simulink library "ddm"  (R2021b)
settings: Solver=VariableStepAuto  StartTime=0.0  StopTime=10.0  RelTol=1e-3
undefined symbols (not defined in the file or in its folder): ENUM_ADASACCSTA_ERROR, ENUM_ADASACCSTA_OFF, ENUM_ADASACCSTA_STANDBY, ENUM_ADASISASTA_OFF, ENUM_ALLOWMOV_ALLOWREADY, ENUM_APS, ENUM_BRKSTA_ERROR, ENUM_BRKSTA_OFF, ENUM_BRKSTA_ON, ENUM_BRKSW_INVALID, ENUM_BRKSW_OFF, ENUM_BRKSW_ON, ENUM_CHGPREACTERRSTA_OBCPRE, ENUM_DCDCFAULTSTA_ANYFAULTLV1, ENUM_DCDCFAULTSTA_ANYFAULTLV2, ENUM_DRIVETRAIN_AWD, ENUM_DRIVETRAIN_FWD, ENUM_DRIVETRAIN_RWD, ENUM_DRSEATSTA_INVALID, ENUM_EDUDRTSTA_NORMAL, ENUM_EPBSTA_APPLIED, ENUM_EPBSTA_RELEASED, ENUM_HVBATTREADYPRE_READY, ENUM_MCUWARN_LV0, ENUM_MCUWARN_LV1, ENUM_MCUWARN_LV2, ENUM_MCUWARN_LV3, ENUM_MCUWARN_NOERROR, ENUM_OBCFAULTSTA_ANYFAULT, ENUM_PAS_R2F2, ENUM_PDFAULT_BATTPDFAIL, ENUM_PDFAULT_DCDCDISABLE, ENUM_PDFAULT_MCUDISABLE, ENUM_PDFAULT_MCUDISCHRG, ENUM_POWERSTA_OFF, ENUM_POWERSTA_ON, ENUM_POWERSTA_READY, ENUM_POWERSTA_STANDBY, ENUM_PRESSINDI_LOW, ENUM_PUFAULT_BATTUPFAIL, ENUM_PUFAULT_DCDCENABLEFAIL, ENUM_PUFAULT_PRECHRGCHKFAIL, ENUM_PUFAULT_SAFETYCHKFAIL, ENUM_PUSTATE_COMPLETED, ENUM_PWRSTASW_OFF, ENUM_PWRSTASW_OFFA, ENUM_PWRSTASW_OFFCHVCHRG, ENUM_PWRSTASW_OFFCLVCHRG, ENUM_PWRSTASW_ON, ENUM_PWRSTASW_ONHVCHRG, ENUM_PWRSTASW_READY, ENUM_PWRSTASW_STANDBY, ENUM_RANGESTA_12IN, ENUM_SHIFTCOMMAND_D, ENUM_SHIFTCOMMAND_N, ENUM_SHIFTCOMMAND_P, ENUM_SHIFTCOMMAND_R, ENUM_VEHMALFUNLV_2ND, ENUM_VEHMALFUNLV_3RD, ENUM_VEHMALFUNLV_4TH ... (+835)
libraries: hcu_lib x750, $bdroot x12, simulink x5
(part 13 of 28)

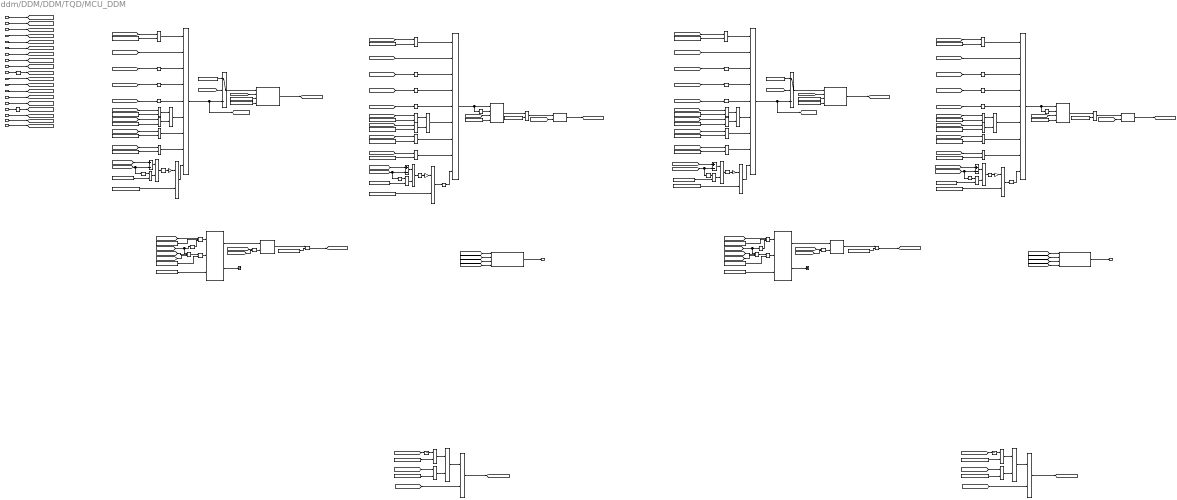
== system ddm/DDM/DDM/TQD/MCU_DDM ==
  note: Front Motor Torque Response Error (FrMCUTqErr)
  note: Fail Safe During Detection
  note: Test Pass Creteria
  note: Test Dtection Criteria
  note: Fail Safe After Detection
  note: Fail Safe During Detection
  note: Test Pass Creteria
  note: Rear Motor Torque Response Error (RrMCUTqErr)
  note: Test Dtection Criteria
  note: Fail Safe After Detection
  task_time_s : Inport
  VPMM_SysPwrSta_enum : Inport  Port=2
  No_CAN3_BUS_OFF : Inport  Port=3
  VDDM_MCUF1NoComCFS_flg : Inport  Port=4
  VDDM_MCUF1RCErrCFS_flg : Inport  Port=5
  VDDM_MCUF1CSErrCFS_flg : Inport  Port=6
  VINP_VehSpeed_kph : Inport  Port=7
  VINP_FrEDUDrtSta_flg : Inport  Port=8
  VINP_FrEDURealTMTq_Nm : Inport  Port=9
  VTQR_FrTMTqReq_Nm : Inport  Port=10
  VDDM_MCUR1NoComCFS_flg : Inport  Port=11
  VDDM_MCUR1RCErrCFS_flg : Inport  Port=12
  VDDM_MCUR1CSErrCFS_flg : Inport  Port=13
  VINP_RrEDUDrtSta_flg : Inport  Port=14
  VINP_RrEDURealTMTq_Nm : Inport  Port=15
  VTQR_RrTMTqReq_Nm : Inport  Port=16
  VINP_MCUWarnF_enum : Inport  Port=17
  VINP_MCUWarnR_enum : Inport  Port=18
  DTC_clear_request : Inport  Port=19
  Abs{,1..7} (8 alike) : Abs
  Add{,1..3} (4 alike) : Sum  Inputs=+-
  Constant{,1,47..48} (4 alike) : Constant  Value=eps
  Constant10 : Constant  Value=ENUM_POWERSTA_OFF
  Constant11 : Constant  Value=ENUM_POWERSTA_STANDBY
  Constant12 : Constant  Value=KDDM_RrMCUTqErrDetSW_flg
  Constant13 : Constant  Value=KDDM_FrMCUTqErrDetSW_flg
  Constant14 : Constant  Value=KDDM_FrMCUTqErrPassSW_flg
  Constant15 : Constant  Value=KDDM_FrMCUTqErrDet_pct
  Constant{4,16,26,32} (4 alike) : Constant  Value=ENUM_MCUWARN_LV0
  Constant{17,27,33,44} (4 alike) : Constant  Value=ENUM_PWRSTASW_OFF
  Constant18 : Constant  Value=ENUM_POWERSTA_OFF
  Constant19 : Constant  Value=ENUM_POWERSTA_STANDBY
  Constant2 : Constant  Value=KDDM_FrMCUTqErrCFSSW_flg
  Constant{5,20,29,34} (4 alike) : Constant  Value=ENUM_MCUWARN_NOERROR
  Constant{6,21,30,35} (4 alike) : Constant  Value=ENUM_EDUDRTSTA_NORMAL
  Constant22 : Constant  Value=KDDM_RrMCUTqErrPassSW_flg
  Constant23 : Constant  Value=KDDM_RrMCUTqErrCFSSW_flg
  Constant24 : Constant  Value=FALSE
  Constant25 : Constant  Value=KDDM_RrMCUTqErrDet_pct
  Constant28 : Constant  Value=KDDM_RrMCUTqErrDTC_cnt
  Constant3 : Constant  Value=KDDM_FrMCUTqErrDet_kph
  Constant31 : Constant  Value=KDDM_RrMCUTqErrDet_kph
  Constant36 : Constant  Value=KDDM_RrMCUTqErrPassTO_s
  Constant37 : Constant  Value=KDDM_RrMCUTqErrDetTO_s
  Constant38 : Constant  Value=KDDM_RrMCUTqErrDet_kph
  Constant39 : Constant  Value=KDDM_RrMCUTqErrPassTO_s
  Constant40 : Constant  Value=KDDM_RrMCUTqErrDTC_cnt
  Constant41 : Constant  Value=KDDM_FrMCUTqErrDet_pct
  Constant42 : Constant  Value=FALSE
  Constant43 : Constant  Value=KDDM_FrMCUTqErrDTC_cnt
  Constant45 : Constant  Value=KDDM_FrMCUTqErrPassTO_s
  Constant46 : Constant  Value=KDDM_FrMCUTqErrDetTO_s
  Constant7 : Constant  Value=KDDM_FrMCUTqErrDet_kph
  Constant70 : Constant  Value=KDDM_FrMCUTqErrPassTO_s
  Constant8 : Constant  Value=KDDM_FrMCUTqErrDTC_cnt
  Constant9 : Constant  Value=KDDM_RrMCUTqErrDet_pct
  DTC_Couter1 : hcu_lib/Basic_Blocks/DTC_Couter
  DTC_Couter2 : hcu_lib/Basic_Blocks/DTC_Couter
  DTC_Info : hcu_lib/Basic_Blocks/DTC_Info
  DTC_Info1 : hcu_lib/Basic_Blocks/DTC_Info
  Divide{,1..3} (4 alike) : Product  Inputs=*/
  Equal{1,3..4,6..10,15..16,21..22,30..31,33..34} (16 alike) : RelationalOperator  Operator===  OutDataTypeStr=boolean  RndMeth=Simplest
  Equal{5,11..12,17..18,27} (6 alike) : RelationalOperator  OutDataTypeStr=boolean  RndMeth=Simplest
  Equal{2,13,19,23} (4 alike) : RelationalOperator  Operator=>  OutDataTypeStr=boolean  RndMeth=Simplest
  Equal{14,20,24,26} (4 alike) : RelationalOperator  Operator=~=  OutDataTypeStr=boolean  RndMeth=Simplest
  Gain{,1..3} (4 alike) : Gain  Gain=100  OutDataTypeStr=single
  Logical Operator{1..2,12,16,20,25,38,40} (8 alike) : Logic  Operator=OR  AllPortsSameDT=off  OutDataTypeStr=boolean
  Logical Operator{3,7,9..10,13..15,17,21..23,26,28,34..37,39} (18 alike) : Logic  Operator=NOT  AllPortsSameDT=off  OutDataTypeStr=boolean
  Logical Operator{11,18,27,30} (4 alike) : Logic  Inputs=9  AllPortsSameDT=off  OutDataTypeStr=boolean
  Logical Operator{4,8,19,24,29,33} (6 alike) : Logic  AllPortsSameDT=off  OutDataTypeStr=boolean
  Logical Operator31 : Logic  Operator=OR  Inputs=3  AllPortsSameDT=off  OutDataTypeStr=boolean
  Logical Operator32 : Logic  Inputs=3  AllPortsSameDT=off  OutDataTypeStr=boolean
  Logical Operator5 : Logic  Operator=OR  Inputs=3  AllPortsSameDT=off  OutDataTypeStr=boolean
  Logical Operator6 : Logic  Inputs=3  AllPortsSameDT=off  OutDataTypeStr=boolean
  Max{,1..3} (4 alike) : MinMax  Function=max  Inputs=2
  Round : Rounding  Operator=round
  Round1 : Rounding  Operator=round
  SR_Latch{1..3,12} (4 alike) : hcu_lib/Basic_Blocks/SR_Latch
  Switch1 : Switch  Criteria=u2 ~= 0
  Switch6 : Switch  Criteria=u2 ~= 0
  Terminator : Terminator
  Terminator1 : Terminator
  Test Detection Criteria1 : hcu_lib/Basic_Blocks/Test Detection Criteria
  Test Detection Criteria2 : hcu_lib/Basic_Blocks/Test Detection Criteria
  Timer1 : hcu_lib/Basic_Blocks/Timer
  Timer2 : hcu_lib/Basic_Blocks/Timer
  Unit Delay : UnitDelay  SampleTime=-1  HasFrameUpgradeWarning=on
  Unit Delay1 : UnitDelay  SampleTime=-1  HasFrameUpgradeWarning=on
  VDDM_FrMCUTqErrDTC_raw32 : Outport
  VDDM_RrMCUTqErrDTC_raw32 : Outport  Port=2
  wires:
  Equal26/1 -> Logical Operator30/1
  Constant44/1 -> Equal26/2
  [VPMM_SysPwrSta_enum] -> Equal26/1
  Logical Operator12/1 -> [VDDM_FrMCUTqErrCFSRls_flg]  "VDDM_FrMCUTqErrCFSRls_flg"
  Constant11/1 -> Equal4/2
  [VPMM_SysPwrSta_enum] -> Unit Delay/1
  [DTC_clear_request] -> Logical Operator12/2
  Equal3/1 -> Logical Operator4/1
  [VPMM_SysPwrSta_enum] -> Equal4/1
  [No_CAN_BUS_OFF] -> Logical Operator30/2
  Equal4/1 -> Logical Operator4/2
  Unit Delay/1 -> Equal3/1
  Logical Operator4/1 -> Logical Operator12/1
  Constant10/1 -> Equal3/2
  Constant3/1 -> Equal2/2
  [VINP_VehSpeed_kph] -> Equal2/1
  Constant4/1 -> Equal6/2
  Constant5/1 -> Equal7/2
  Equal6/1 -> Logical Operator1/1
  Equal7/1 -> Logical Operator1/2
  Logical Operator1/1 -> Logical Operator30/6
  [VINP_FrEDUDrtSta_flg] -> Equal10/1
  Constant6/1 -> Equal10/2
  Equal10/1 -> Logical Operator30/7
  Equal2/1 -> Logical Operator30/8
  [VDDM_MCUF1CSErrCFS_flg] -> Logical Operator10/1
  [VDDM_MCUF1RCErrCFS_flg] -> Logical Operator9/1
  Logical Operator9/1 -> Logical Operator30/4
  [VDDM_MCUF1NoComCFS_flg] -> Logical Operator7/1
  Logical Operator7/1 -> Logical Operator30/3
  Logical Operator10/1 -> Logical Operator30/5
  Add/1 -> Divide/1
  Abs/1 -> Gain/1
  Divide/1 -> Abs/1
  [VINP_FrEDURealTMTq_Nm] -> Add/1
  [VTQR_FrTMTqReq_Nm] -> Abs4/1, Add/2
  Gain/1 -> Equal12/1
  Equal12/1 -> Logical Operator30/9
  Constant15/1 -> Equal12/2
  Logical Operator2/1 -> Logical Operator11/6
  [VINP_FrEDUDrtSta_flg] -> Equal1/1
  Constant20/1 -> Equal16/2
  [VDDM_MCUF1NoComCFS_flg] -> Logical Operator13/1
  Equal1/1 -> Logical Operator11/7
  Constant16/1 -> Equal15/2
  Equal13/1 -> Logical Operator11/8
  Logical Operator14/1 -> Logical Operator11/4
  [VDDM_MCUF1RCErrCFS_flg] -> Logical Operator14/1
  Constant7/1 -> Equal13/2
  Constant21/1 -> Equal1/2
  [VINP_VehSpeed_kph] -> Equal13/1
  Logical Operator3/1 -> Logical Operator11/5
  [VDDM_MCUF1CSErrCFS_flg] -> Logical Operator3/1
  Constant17/1 -> Equal14/2
  [No_CAN_BUS_OFF] -> Logical Operator11/2
  Equal16/1 -> Logical Operator2/2
  [VPMM_SysPwrSta_enum] -> Equal14/1
  Equal14/1 -> Logical Operator11/1
  Equal15/1 -> Logical Operator2/1
  Logical Operator13/1 -> Logical Operator11/3
  Equal11/1 -> Logical Operator15/1
  Logical Operator15/1 -> Logical Operator11/9
  [VDDM_MCUR1CSErrCFS_flg] -> Logical Operator17/1
  Equal8/1 -> Logical Operator18/7
  Logical Operator22/1 -> Logical Operator18/4
  [VDDM_MCUR1RCErrCFS_flg] -> Logical Operator22/1
  Equal33/1 -> Logical Operator16/1
  [VINP_MCUWarnR_enum] -> Equal33/1
  [VINP_VehSpeed_kph] -> Equal23/1
  Constant38/1 -> Equal19/2
  [VDDM_MCUR1CSErrCFS_flg] -> Logical Operator26/1
  Constant27/1 -> Equal20/2
  Logical Operator21/1 -> Logical Operator18/3
  Equal21/1 -> Logical Operator25/1
  Logical Operator26/1 -> Logical Operator18/5
  [VINP_VehSpeed_kph] -> Equal19/1
  Constant18/1 -> Equal30/2
  [VPMM_SysPwrSta_enum] -> Equal20/1
  [No_CAN_BUS_OFF] -> Logical Operator18/2
  Logical Operator23/1 -> Logical Operator18/9
  Logical Operator29/1 -> Logical Operator20/1
  Equal20/1 -> Logical Operator18/1
  [VINP_MCUWarnR_enum] -> Equal34/1
  Logical Operator17/1 -> Logical Operator27/5
  Equal34/1 -> Logical Operator16/2
  Equal31/1 -> Logical Operator29/2
  [VPMM_SysPwrSta_enum] -> Equal31/1
  Equal18/1 -> Logical Operator27/9
  [VDDM_MCUR1NoComCFS_flg] -> Logical Operator35/1
  Equal22/1 -> Logical Operator25/2
  Constant33/1 -> Equal24/2
  Equal23/1 -> Logical Operator27/8
  Constant26/1 -> Equal21/2
  Equal19/1 -> Logical Operator18/8
  Equal9/1 -> Logical Operator27/7
  Unit Delay1/1 -> Equal30/1
  [VDDM_MCUR1RCErrCFS_flg] -> Logical Operator37/1
  Constant30/1 -> Equal8/2
  Constant29/1 -> Equal22/2
  [VDDM_MCUR1NoComCFS_flg] -> Logical Operator21/1
  Constant35/1 -> Equal9/2
  Logical Operator35/1 -> Logical Operator27/3
  Constant32/1 -> Equal33/2
  [VINP_RrEDUDrtSta_flg] -> Equal9/1
  Constant34/1 -> Equal34/2
  [No_CAN_BUS_OFF] -> Logical Operator27/2
  [VPMM_SysPwrSta_enum] -> Unit Delay1/1
  Equal30/1 -> Logical Operator29/1
  Constant31/1 -> Equal23/2
  Logical Operator25/1 -> Logical Operator18/6
  Constant19/1 -> Equal31/2
  [DTC_clear_request] -> Logical Operator20/2
  Logical Operator16/1 -> Logical Operator27/6
  Equal24/1 -> Logical Operator27/1
  [VPMM_SysPwrSta_enum] -> Equal24/1
  [VINP_RrEDUDrtSta_flg] -> Equal8/1
  Logical Operator37/1 -> Logical Operator27/4
  Logical Operator20/1 -> [VDDM_RrMCUTqErrCFSRls_flg]  "VDDM_RrMCUTqErrCFSRls_flg"
  Logical Operator11/1 -> Logical Operator34/1, Timer1/1
  [task_time_s] -> Test Detection Criteria1/2
  [task_time_s] -> Timer1/3
  Constant42/1 -> Switch6/1
  Test Detection Criteria1/1 -> [VDDM_FrMCUTqErrDet_flg]  "VDDM_FrMCUTqErrDet_flg"
  Equal27/1 -> SR_Latch12/1
  Logical Operator34/1 -> Timer1/2
  Timer1/1 -> Equal27/1
  Constant43/1 -> Test Detection Criteria1/3
  Switch6/1 -> Test Detection Criteria1/1
  SR_Latch12/1 -> [VDDM_FrMCUTqErrPass_flg]  "VDDM_FrMCUTqErrPass_flg"
  Logical Operator30/1 -> [VDDM_FrMCUTqErrRst_flg], Switch6/3
  Constant46/1 -> Test Detection Criteria1/4
  Constant70/1 -> Timer1/4
  Constant45/1 -> Equal27/2
  [VDDM_FrMCUTqErrRst_flg] -> SR_Latch12/2
  [DTC_clear_request] -> Switch6/2
  [VDDM_FrMCUTqErrDet_flg] -> DTC_Info/1
  Logical Operator19/1 -> [VDDM_FrMCUTqErrCFS_flg]  "VDDM_FrMCUTqErrCFS_flg"
  [VDDM_FrMCUTqErrCFSRls_flg] -> Logical Operator38/1
  DTC_Info/1 -> VDDM_FrMCUTqErrDTC_raw32/1  "VDDM_FrMCUTqErrDTC_raw32"
  [VDDM_FrMCUTqErrCFSRls_flg] -> Logical Operator5/3
  DTC_Couter1/1 -> SR_Latch1/1
  [VDDM_FrMCUTqErrPass_flg] -> Logical Operator5/2
  Constant13/1 -> Logical Operator6/2
  Logical Operator5/1 -> Logical Operator8/1
  [DTC_clear_request] -> DTC_Info/4
  Logical Operator6/1 -> DTC_Couter1/1
  Logical Operator8/1 -> DTC_Couter1/2
  SR_Latch1/1 -> Logical Operator19/1
  [VDDM_FrMCUTqErrDet_flg] -> Logical Operator6/1
  Constant2/1 -> Logical Operator19/2
  Constant14/1 -> Logical Operator8/2
  [VDDM_FrMCUTqErrCFS_flg] -> DTC_Info/3
  Constant8/1 -> DTC_Couter1/3
  [VDDM_FrMCUTqErrPass_flg] -> DTC_Info/2
  DTC_Couter1/2 -> Terminator/1
  DTC_Couter2/1 -> SR_Latch2/1
  [DTC_clear_request] -> Switch1/2
  [VDDM_RrMCUTqErrCFSRls_flg] -> Logical Operator31/3
  [VDDM_RrMCUTqErrCFSRls_flg] -> Logical Operator40/1
  Test Detection Criteria2/1 -> [VDDM_RrMCUTqErrDet_flg]  "VDDM_RrMCUTqErrDet_flg"
  [VDDM_RrMCUTqErrDet_flg] -> DTC_Info1/1
  Constant12/1 -> Logical Operator32/2
  DTC_Info1/1 -> VDDM_RrMCUTqErrDTC_raw32/1  "VDDM_RrMCUTqErrDTC_raw32"
  [DTC_clear_request] -> DTC_Info1/4
  SR_Latch3/1 -> [VDDM_RrMCUTqErrPass_flg]  "VDDM_RrMCUTqErrPass_flg"
  Logical Operator24/1 -> [VDDM_RrMCUTqErrCFS_flg]  "VDDM_RrMCUTqErrCFS_flg"
  Constant22/1 -> Logical Operator33/2
  Constant23/1 -> Logical Operator24/2
  [VDDM_RrMCUTqErrCFS_flg] -> DTC_Info1/3
  SR_Latch2/1 -> Logical Operator24/1
  Constant39/1 -> Timer2/4
  Logical Operator32/1 -> DTC_Couter2/1
  Logical Operator33/1 -> DTC_Couter2/2
  [VDDM_RrMCUTqErrPass_flg] -> Logical Operator31/2
  DTC_Couter2/2 -> Terminator1/1
  Logical Operator31/1 -> Logical Operator33/1
  Constant24/1 -> Switch1/1
  [task_time_s] -> Timer2/3
  Timer2/1 -> Equal5/1
  Constant40/1 -> DTC_Couter2/3
  [VDDM_RrMCUTqErrPass_flg] -> DTC_Info1/2
  [task_time_s] -> Test Detection Criteria2/2
  Equal5/1 -> SR_Latch3/1
  Constant28/1 -> Test Detection Criteria2/3
  Logical Operator27/1 -> [VDDM_RrMCUTqErrRst_flg], Switch1/3
  Constant37/1 -> Test Detection Criteria2/4
  [VDDM_RrMCUTqErrRst_flg] -> SR_Latch3/2
  Switch1/1 -> Test Detection Criteria2/1
  [VDDM_RrMCUTqErrDet_flg] -> Logical Operator32/1
  Logical Operator28/1 -> Timer2/2
  Constant36/1 -> Equal5/2
  Logical Operator18/1 -> Logical Operator28/1, Timer2/1
  task_time_s/1 -> [task_time_s]
  VPMM_SysPwrSta_enum/1 -> [VPMM_SysPwrSta_enum]
  No_CAN3_BUS_OFF/1 -> [No_CAN_BUS_OFF]
  VDDM_MCUF1NoComCFS_flg/1 -> [VDDM_MCUF1NoComCFS_flg]
  VDDM_MCUF1RCErrCFS_flg/1 -> [VDDM_MCUF1RCErrCFS_flg]
  VDDM_MCUF1CSErrCFS_flg/1 -> [VDDM_MCUF1CSErrCFS_flg]
  VINP_FrEDUDrtSta_flg/1 -> [VINP_FrEDUDrtSta_flg]
  VINP_VehSpeed_kph/1 -> [VINP_VehSpeed_kph]
  VTQR_FrTMTqReq_Nm/1 -> Round1/1
  VDDM_MCUR1NoComCFS_flg/1 -> [VDDM_MCUR1NoComCFS_flg]
  VDDM_MCUR1RCErrCFS_flg/1 -> [VDDM_MCUR1RCErrCFS_flg]
  VDDM_MCUR1CSErrCFS_flg/1 -> [VDDM_MCUR1CSErrCFS_flg]
  VINP_RrEDUDrtSta_flg/1 -> [VINP_RrEDUDrtSta_flg]
  VTQR_RrTMTqReq_Nm/1 -> Round/1
  DTC_clear_request/1 -> [DTC_clear_request]
  VINP_MCUWarnF_enum/1 -> [VINP_MCUWarnF_enum]
  VINP_MCUWarnR_enum/1 -> [VINP_MCUWarnR_enum]
  [VINP_MCUWarnF_enum] -> Equal6/1
  [VINP_MCUWarnF_enum] -> Equal7/1
  [VINP_MCUWarnF_enum] -> Equal15/1
  [VINP_MCUWarnF_enum] -> Equal16/1
  [VINP_MCUWarnR_enum] -> Equal21/1
  [VINP_MCUWarnR_enum] -> Equal22/1
  Constant/1 -> Max/2
  Abs4/1 -> Max/1
  Max/1 -> Divide/2
  Max1/1 -> Divide1/2
  Constant1/1 -> Max1/2
  Abs1/1 -> Gain1/1
  Gain1/1 -> Equal11/1
  Add1/1 -> Divide1/1
  Constant41/1 -> Equal11/2
  Abs5/1 -> Max1/1
  Divide1/1 -> Abs1/1
  [VINP_FrEDURealTMTq_Nm] -> Add1/1
  [VTQR_FrTMTqReq_Nm] -> Abs5/1, Add1/2
  Abs6/1 -> Max2/1
  Abs2/1 -> Gain2/1
  Max2/1 -> Divide2/2
  Constant47/1 -> Max2/2
  Constant25/1 -> Equal18/2
  Divide2/1 -> Abs2/1
  Add2/1 -> Divide2/1
  Gain2/1 -> Equal18/1
  Gain3/1 -> Equal17/1
  Max3/1 -> Divide3/2
  Abs7/1 -> Max3/1
  Divide3/1 -> Abs3/1
  Constant48/1 -> Max3/2
  Constant9/1 -> Equal17/2
  Add3/1 -> Divide3/1
  Abs3/1 -> Gain3/1
  Equal17/1 -> Logical Operator23/1
  Logical Operator36/1 -> Logical Operator6/3
  [DTC_clear_request] -> Logical Operator5/1, Logical Operator36/1
  Logical Operator38/1 -> SR_Latch1/2
  [DTC_clear_request] -> Logical Operator38/2
  [DTC_clear_request] -> Logical Operator31/1, Logical Operator39/1
  Logical Operator39/1 -> Logical Operator32/3
  Logical Operator40/1 -> SR_Latch2/2
  [DTC_clear_request] -> Logical Operator40/2
  [VINP_RrEDURealTMTq_Nm] -> Add2/1
  [VTQR_RrTMTqReq_Nm] -> Abs6/1, Add2/2
  [VINP_RrEDURealTMTq_Nm] -> Add3/1
  [VTQR_RrTMTqReq_Nm] -> Abs7/1, Add3/2
  Round/1 -> [VTQR_RrTMTqReq_Nm]
  VINP_RrEDURealTMTq_Nm/1 -> [VINP_RrEDURealTMTq_Nm]
  Round1/1 -> [VTQR_FrTMTqReq_Nm]
  VINP_FrEDURealTMTq_Nm/1 -> [VINP_FrEDURealTMTq_Nm]

== system ddm/DDM/DDM/TQD/Shifter1_DDM ==
  note: Shifter1 Lost Comm (Shifter1NoCom)
  note: Shifter1 Rolling Count Error (Shifter1RCErr)
  note: Shifter1 Rolling Count Error (Shifter1CSErr)
  task_time_s : Inport
  VPMM_SysPwrSta_enum : Inport  Port=2
  No_CAN3_BUS_OFF : Inport  Port=3
  VDDM_Shifter1NoCom_flg : Inport  Port=4
  VDDM_Shifter1RCErr_flg : Inport  Port=5
  VDDM_Shifter1CSErr_flg : Inport  Port=6
  DTC_clear_request : Inport  Port=7
  Constant1 : Constant  Value=KDDM_Shifter1NoComCFSSW_flg
  Constant10 : Constant  Value=KDDM_Shifter1RCErrDFSSW_flg
  Constant{3,11,17,19,31,36} (6 alike) : Constant  Value=ENUM_PWRSTASW_OFF
  Constant12 : Constant  Value=FALSE
  Constant13 : Constant  Value=KDDM_Shifter1RCErrDTC_cnt
  Constant14 : Constant  Value=KDDM_Shifter1RCErrPassTO_s
  Constant15 : Constant  Value=KDDM_Shifter1NoComDTC_cnt
  Constant16 : Constant  Value=KDDM_Shifter1NoComDFSSW_flg
  Constant18 : Constant  Value=KDDM_Shifter1RCErrDetTO_s
  Constant2 : Constant  Value=FALSE
  Constant20 : Constant  Value=KDDM_Shifter1NoComDTC_cnt
  Constant21 : Constant  Value=KDDM_Shifter1NoComPassTO_s
  Constant22 : Constant  Value=KDDM_Shifter1NoComDetTO_s
  Constant23 : Constant  Value=ENUM_POWERSTA_OFF
  Constant24 : Constant  Value=ENUM_POWERSTA_STANDBY
  Constant25 : Constant  Value=KDDM_Shifter1RCErrDetSW_flg
  Constant26 : Constant  Value=KDDM_Shifter1RCErrPassSW_flg
  Constant27 : Constant  Value=KDDM_Shifter1RCErrPassTO_s
  Constant28 : Constant  Value=KDDM_Shifter1CSErrCFSSW_flg
  Constant29 : Constant  Value=KDDM_Shifter1CSErrDTC_cnt
  Constant30 : Constant  Value=KDDM_Shifter1CSErrDFSSW_flg
  Constant32 : Constant  Value=FALSE
  Constant33 : Constant  Value=KDDM_Shifter1CSErrDTC_cnt
  Constant34 : Constant  Value=KDDM_Shifter1CSErrPassTO_s
  Constant35 : Constant  Value=KDDM_Shifter1CSErrDetTO_s
  Constant37 : Constant  Value=ENUM_POWERSTA_OFF
  Constant38 : Constant  Value=ENUM_POWERSTA_STANDBY
  Constant39 : Constant  Value=KDDM_Shifter1CSErrDetSW_flg
  Constant4 : Constant  Value=ENUM_POWERSTA_OFF
  Constant40 : Constant  Value=KDDM_Shifter1CSErrPassSW_flg
  Constant41 : Constant  Value=KDDM_Shifter1CSErrPassTO_s
  Constant5 : Constant  Value=ENUM_POWERSTA_STANDBY
  Constant6 : Constant  Value=KDDM_Shifter1NoComDetSW_flg
  Constant7 : Constant  Value=KDDM_Shifter1NoComPassSW_flg
  Constant70 : Constant  Value=KDDM_Shifter1NoComPassTO_s
  Constant8 : Constant  Value=KDDM_Shifter1RCErrCFSSW_flg
  Constant9 : Constant  Value=KDDM_Shifter1RCErrDTC_cnt
  DTC_Couter1 : hcu_lib/Basic_Blocks/DTC_Couter
  DTC_Couter2 : hcu_lib/Basic_Blocks/DTC_Couter
  DTC_Couter3 : hcu_lib/Basic_Blocks/DTC_Couter
  DTC_Info : hcu_lib/Basic_Blocks/DTC_Info
  DTC_Info1 : hcu_lib/Basic_Blocks/DTC_Info
  DTC_Info2 : hcu_lib/Basic_Blocks/DTC_Info
  Data Type Conversion1 : DataTypeConversion  OutDataTypeStr=uint8
  Data Type Conversion2 : DataTypeConversion  OutDataTypeStr=uint8
  Data Type Conversion3 : DataTypeConversion  OutDataTypeStr=uint8
  Equal{1,3,9..12} (6 alike) : RelationalOperator  Operator===  OutDataTypeStr=boolean  RndMeth=Simplest
  Equal{2,4..6,13..14} (6 alike) : RelationalOperator  Operator=~=  OutDataTypeStr=boolean  RndMeth=Simplest
  Equal15 : RelationalOperator  OutDataTypeStr=boolean  RndMeth=Simplest
  Equal7 : RelationalOperator  OutDataTypeStr=boolean  RndMeth=Simplest
  Equal8 : RelationalOperator  OutDataTypeStr=boolean  RndMeth=Simplest
  Logical Operator{1,3,25,40,42,44} (6 alike) : Logic  Operator=OR  AllPortsSameDT=off  OutDataTypeStr=boolean
  Logical Operator{7,10,15,17,31} (5 alike) : Logic  Inputs=3  AllPortsSameDT=off  OutDataTypeStr=boolean
  Logical Operator{5,11,23,27,37,77} (6 alike) : Logic  Operator=OR  Inputs=3  AllPortsSameDT=off  OutDataTypeStr=boolean
  Logical Operator{6,9,12,14,20,24,28,30,34,38..39,41,43} (13 alike) : Logic  Operator=NOT  AllPortsSameDT=off  OutDataTypeStr=boolean
  Logical Operator{2,8,13,16,18..19,21,29,32..33,35,55} (12 alike) : Logic  AllPortsSameDT=off  OutDataTypeStr=boolean
  Logical Operator{4,22,26,36} (4 alike) : Logic  Inputs=4  AllPortsSameDT=off  OutDataTypeStr=boolean
  Relay1 : Relay  OnSwitchValue=ONE_INT  OffSwitchValue=ZERO_INT
  Relay2 : Relay  OnSwitchValue=ONE_INT  OffSwitchValue=ZERO_INT
  Relay3 : Relay  OnSwitchValue=ONE_INT  OffSwitchValue=ZERO_INT
  SR_Latch{1..8,12} (9 alike) : hcu_lib/Basic_Blocks/SR_Latch
  Switch1 : Switch  Criteria=u2 ~= 0
  Switch2 : Switch  Criteria=u2 ~= 0
  Switch6 : Switch  Criteria=u2 ~= 0
  Test Detection Criteria1 : hcu_lib/Basic_Blocks/Test Detection Criteria
  Test Detection Criteria2 : hcu_lib/Basic_Blocks/Test Detection Criteria
  Test Detection Criteria3 : hcu_lib/Basic_Blocks/Test Detection Criteria
  Timer1 : hcu_lib/Basic_Blocks/Timer
  Timer2 : hcu_lib/Basic_Blocks/Timer
  Timer3 : hcu_lib/Basic_Blocks/Timer
  Unit Delay1 : UnitDelay  SampleTime=-1  HasFrameUpgradeWarning=on
  Unit Delay2 : UnitDelay  SampleTime=-1  HasFrameUpgradeWarning=on
  Unit Delay3 : UnitDelay  SampleTime=-1  HasFrameUpgradeWarning=on
  VDDM_Shifter1NoComDTC_raw32 : Outport
  VDDM_Shifter1RCErrDTC_raw32 : Outport  Port=2
  VDDM_Shifter1CSErrDTC_raw32 : Outport  Port=3
  VDDM_Shifter1NoComCFS_flg : Outport  Port=4
  VDDM_Shifter1RCErrCFS_flg : Outport  Port=5
  VDDM_Shifter1CSErrCFS_flg : Outport  Port=6
  wires:
  Logical Operator77/1 -> SR_Latch2/2
  [DTC_clear_request] -> Logical Operator1/2
  SR_Latch2/1 -> Logical Operator55/2
  Logical Operator14/1 -> Timer2/2
  [VDDM_Shifter1NoComCFSRls_flg] -> Logical Operator40/1
  Logical Operator13/1 -> Logical Operator1/1
  Relay1/1 -> SR_Latch2/1
  Constant22/1 -> Test Detection Criteria1/4
  Logical Operator16/1 -> DTC_Couter1/2
  Logical Operator7/1 -> Logical Operator14/1, Timer2/1
  Timer2/1 -> Equal7/1
  Equal10/1 -> Logical Operator13/1
  SR_Latch12/1 -> [VDDM_Shifter1NoComPass_flg]  "VDDM_Shifter1NoComPass_flg"
  DTC_Couter1/2 -> Data Type Conversion2/1
  Constant4/1 -> Equal10/2
  [VDDM_Shifter1NoComDet_flg] -> Logical Operator15/1
  Constant6/1 -> Logical Operator15/2
  Test Detection Criteria1/1 -> [VDDM_Shifter1NoComDet_flg]  "VDDM_Shifter1NoComDet_flg"
  Logical Operator15/1 -> DTC_Couter1/1
  [VDDM_Shifter1NoComCFSRls_flg] -> Logical Operator11/3
  [VDDM_Shifter1NoComDFSRls_flg] -> Logical Operator77/1
  [VDDM_Shifter1NoComPass_flg] -> Logical Operator11/2
  [VDDM_Shifter1NoComDTC_cnt] -> Relay1/1
  Constant20/1 -> Test Detection Criteria1/3
  [VDDM_Shifter1NoComCFS_flg] -> Logical Operator77/2
  [VPMM_SysPwrSta_enum] -> Equal11/1
  Equal7/1 -> SR_Latch12/1
  Equal11/1 -> Logical Operator13/2
  Unit Delay2/1 -> Equal10/1
  Logical Operator11/1 -> Logical Operator16/1
  Constant16/1 -> Logical Operator55/1
  Data Type Conversion2/1 -> [VDDM_Shifter1NoComDTC_cnt]  "VDDM_Shifter1NoComDTC_cnt"
  Logical Operator55/1 -> [VDDM_Shifter1NoComDFS_flg]  "VDDM_Shifter1NoComDFS_flg"
  Constant15/1 -> DTC_Couter1/3
  Constant5/1 -> Equal11/2
  Constant7/1 -> Logical Operator16/2
  Logical Operator1/1 -> [VDDM_Shifter1NoComCFSRls_flg]  "VDDM_Shifter1NoComCFSRls_flg"
  Constant70/1 -> Timer2/4
  DTC_Couter1/1 -> SR_Latch1/1
  [VPMM_SysPwrSta_enum] -> Unit Delay2/1
  [task_time_s] -> Test Detection Criteria1/2
  Constant21/1 -> Equal7/2
  [task_time_s] -> Timer2/3
  [No_CAN3_BUS_OFF] -> Logical Operator10/2
  Equal6/1 -> Logical Operator10/1
  Constant17/1 -> Equal6/2
  [VDDM_Shifter1NoCom_flg] -> Logical Operator10/3
  [VPMM_SysPwrSta_enum] -> Equal6/1
  [VDDM_Shifter1NoCom_flg] -> Logical Operator9/1
  Equal2/1 -> Logical Operator7/1
  Logical Operator9/1 -> Logical Operator7/3
  Constant3/1 -> Equal2/2
  [No_CAN3_BUS_OFF] -> Logical Operator7/2
  [VPMM_SysPwrSta_enum] -> Equal2/1
  VDDM_Shifter1NoCom_flg/1 -> [VDDM_Shifter1NoCom_flg]
  VPMM_SysPwrSta_enum/1 -> [VPMM_SysPwrSta_enum]
  [VDDM_Shifter1NoComCFS_flg] -> DTC_Info/3
  DTC_Info/1 -> VDDM_Shifter1NoComDTC_raw32/1  "VDDM_Shifter1NoComDTC_raw32"
  [VDDM_Shifter1NoComPass_flg] -> DTC_Info/2
  task_time_s/1 -> [task_time_s]
  DTC_clear_request/1 -> [DTC_clear_request]
  [VDDM_Shifter1NoComDet_flg] -> DTC_Info/1
  No_CAN3_BUS_OFF/1 -> [No_CAN3_BUS_OFF]
  Constant1/1 -> Logical Operator2/2
  Logical Operator2/1 -> [VDDM_Shifter1NoComCFS_flg]  "VDDM_Shifter1NoComCFS_flg"
  SR_Latch1/1 -> Logical Operator2/1
  [DTC_clear_request] -> DTC_Info/4
  [DTC_clear_request] -> Switch6/2
  Switch6/1 -> Test Detection Criteria1/1
  Logical Operator10/1 -> [VDDM_Shifter1NoComRst_flg], Switch6/3
  Constant2/1 -> Switch6/1
  Logical Operator20/1 -> Logical Operator4/4
  [DTC_clear_request] -> Logical Operator3/2
  Constant26/1 -> Logical Operator18/2
  Logical Operator12/1 -> Timer1/2
  SR_Latch5/1 -> Logical Operator21/2
  [VPMM_SysPwrSta_enum] -> Equal4/1
  [VDDM_Shifter1RCErrPass_flg] -> Logical Operator5/2
  Logical Operator8/1 -> Logical Operator3/1
  Logical Operator19/1 -> [VDDM_Shifter1RCErrCFS_flg]  "VDDM_Shifter1RCErrCFS_flg"
  Constant13/1 -> Test Detection Criteria2/3
  Equal1/1 -> Logical Operator8/1
  Constant25/1 -> Logical Operator17/2
  Logical Operator5/1 -> Logical Operator18/1
  SR_Latch4/1 -> [VDDM_Shifter1RCErrPass_flg]  "VDDM_Shifter1RCErrPass_flg"
  Logical Operator17/1 -> DTC_Couter2/1
  [VDDM_Shifter1RCErrCFS_flg] -> Logical Operator23/2
  DTC_Couter2/2 -> Data Type Conversion1/1
  Equal5/1 -> Logical Operator4/1
  Logical Operator22/1 -> Timer1/1, Logical Operator12/1
  Unit Delay1/1 -> Equal1/1
  [VDDM_Shifter1NoComCFS_flg] -> Logical Operator20/1
  Constant24/1 -> Equal3/2
  Logical Operator21/1 -> [VDDM_Shifter1RCErrDFS_flg]  "VDDM_Shifter1RCErrDFS_flg"
  Constant14/1 -> Equal8/2
  [VDDM_Shifter1RCErr_flg] -> Logical Operator24/1
  Logical Operator3/1 -> [VDDM_Shifter1RCErrCFSRls_flg]  "VDDM_Shifter1RCErrCFSRls_flg"
  Constant19/1 -> Equal4/2
  Equal8/1 -> SR_Latch4/1
  [VDDM_Shifter1RCErrCFSRls_flg] -> Logical Operator42/1
  Constant11/1 -> Equal5/2
  Constant18/1 -> Test Detection Criteria2/4
  [VDDM_Shifter1RCErrPass_flg] -> DTC_Info1/2
  [No_CAN3_BUS_OFF] -> Logical Operator22/2
  Equal4/1 -> Logical Operator22/1
  Constant23/1 -> Equal1/2
  Logical Operator18/1 -> DTC_Couter2/2
  Data Type Conversion1/1 -> [VDDM_Shifter1RCErrDTC_cnt]  "VDDM_Shifter1RCErrDTC_cnt"
  DTC_Info1/1 -> VDDM_Shifter1RCErrDTC_raw32/1  "VDDM_Shifter1RCErrDTC_raw32"
  Constant10/1 -> Logical Operator21/1
  Logical Operator23/1 -> SR_Latch5/2
  [VPMM_SysPwrSta_enum] -> Equal3/1
  [VPMM_SysPwrSta_enum] -> Equal5/1
  [No_CAN3_BUS_OFF] -> Logical Operator4/2
  [VDDM_Shifter1RCErrDet_flg] -> DTC_Info1/1
  Relay2/1 -> SR_Latch5/1
  [VDDM_Shifter1RCErrDet_flg] -> Logical Operator17/1
  [task_time_s] -> Timer1/3
  [task_time_s] -> Test Detection Criteria2/2
  Constant27/1 -> Timer1/4
  Timer1/1 -> Equal8/1
  SR_Latch3/1 -> Logical Operator19/1
  [DTC_clear_request] -> Switch1/2
  Constant12/1 -> Switch1/1
  Equal3/1 -> Logical Operator8/2
  [VDDM_Shifter1RCErrDTC_cnt] -> Relay2/1
  [VDDM_Shifter1RCErrCFS_flg] -> DTC_Info1/3
  [VPMM_SysPwrSta_enum] -> Unit Delay1/1
  Constant9/1 -> DTC_Couter2/3
  Logical Operator4/1 -> [VDDM_Shifter1RCErrRst_flg], Switch1/3
  [VDDM_Shifter1RCErrDFSRls_flg] -> Logical Operator23/1
  [VDDM_Shifter1RCErrCFSRls_flg] -> Logical Operator5/3
  Logical Operator24/1 -> Logical Operator22/3
  DTC_Couter2/1 -> SR_Latch3/1
  [DTC_clear_request] -> DTC_Info1/4
  Constant8/1 -> Logical Operator19/2
  [VDDM_Shifter1RCErr_flg] -> Logical Operator4/3
  Test Detection Criteria2/1 -> [VDDM_Shifter1RCErrDet_flg]  "VDDM_Shifter1RCErrDet_flg"
  Logical Operator34/1 -> Logical Operator26/4
  [DTC_clear_request] -> Logical Operator25/2
  Constant40/1 -> Logical Operator32/2
  Logical Operator30/1 -> Timer3/2
  SR_Latch8/1 -> Logical Operator35/2
  [VPMM_SysPwrSta_enum] -> Equal13/1
  [VDDM_Shifter1CSErrPass_flg] -> Logical Operator27/2
  Logical Operator29/1 -> Logical Operator25/1
  Logical Operator33/1 -> [VDDM_Shifter1CSErrCFS_flg]  "VDDM_Shifter1CSErrCFS_flg"
  Constant33/1 -> Test Detection Criteria3/3
  Equal9/1 -> Logical Operator29/1
  Constant39/1 -> Logical Operator31/2
  Logical Operator27/1 -> Logical Operator32/1
  SR_Latch7/1 -> [VDDM_Shifter1CSErrPass_flg]  "VDDM_Shifter1CSErrPass_flg"
  Logical Operator31/1 -> DTC_Couter3/1
  [VDDM_Shifter1CSErrCFS_flg] -> Logical Operator37/2
  DTC_Couter3/2 -> Data Type Conversion3/1
  Equal14/1 -> Logical Operator26/1
  Logical Operator36/1 -> Timer3/1, Logical Operator30/1
  Unit Delay3/1 -> Equal9/1
  [VDDM_Shifter1NoComCFS_flg] -> Logical Operator34/1
  Constant38/1 -> Equal12/2
  Logical Operator35/1 -> [VDDM_Shifter1CSErrDFS_flg]  "VDDM_Shifter1CSErrDFS_flg"
  Constant34/1 -> Equal15/2
  [VDDM_Shifter1CSErr_flg] -> Logical Operator38/1
  Logical Operator25/1 -> [VDDM_Shifter1CSErrCFSRls_flg]  "VDDM_Shifter1CSErrCFSRls_flg"
  Constant36/1 -> Equal13/2
  Equal15/1 -> SR_Latch7/1
  [VDDM_Shifter1CSErrCFSRls_flg] -> Logical Operator44/1
  Constant31/1 -> Equal14/2
  Constant35/1 -> Test Detection Criteria3/4
  [VDDM_Shifter1CSErrPass_flg] -> DTC_Info2/2
  [No_CAN3_BUS_OFF] -> Logical Operator36/2
  Equal13/1 -> Logical Operator36/1
  Constant37/1 -> Equal9/2
  Logical Operator32/1 -> DTC_Couter3/2
  Data Type Conversion3/1 -> [VDDM_Shifter1CSErrDTC_cnt]  "VDDM_Shifter1CSErrDTC_cnt"
  DTC_Info2/1 -> VDDM_Shifter1CSErrDTC_raw32/1  "VDDM_Shifter1CSErrDTC_raw32"
  Constant30/1 -> Logical Operator35/1
  Logical Operator37/1 -> SR_Latch8/2
  [VPMM_SysPwrSta_enum] -> Equal12/1
  [VPMM_SysPwrSta_enum] -> Equal14/1
  [No_CAN3_BUS_OFF] -> Logical Operator26/2
  [VDDM_Shifter1CSErrDet_flg] -> DTC_Info2/1
  Relay3/1 -> SR_Latch8/1
  [VDDM_Shifter1CSErrDet_flg] -> Logical Operator31/1
  [task_time_s] -> Timer3/3
  [task_time_s] -> Test Detection Criteria3/2
  Constant41/1 -> Timer3/4
  Timer3/1 -> Equal15/1
  SR_Latch6/1 -> Logical Operator33/1
  [DTC_clear_request] -> Switch2/2
  Constant32/1 -> Switch2/1
  Equal12/1 -> Logical Operator29/2
  [VDDM_Shifter1CSErrDTC_cnt] -> Relay3/1
  [VDDM_Shifter1CSErrCFS_flg] -> DTC_Info2/3
  [VPMM_SysPwrSta_enum] -> Unit Delay3/1
  Constant29/1 -> DTC_Couter3/3
  Logical Operator26/1 -> [VDDM_Shifter1CSErrRst_flg], Switch2/3
  [VDDM_Shifter1CSErrDFSRls_flg] -> Logical Operator37/1
  [VDDM_Shifter1CSErrCFSRls_flg] -> Logical Operator27/3
  Logical Operator38/1 -> Logical Operator36/3
  DTC_Couter3/1 -> SR_Latch6/1
  [DTC_clear_request] -> DTC_Info2/4
  Constant28/1 -> Logical Operator33/2
  [VDDM_Shifter1CSErr_flg] -> Logical Operator26/3
  Test Detection Criteria3/1 -> [VDDM_Shifter1CSErrDet_flg]  "VDDM_Shifter1CSErrDet_flg"
  [VDDM_Shifter1NoComRst_flg] -> SR_Latch12/2
  Switch1/1 -> Test Detection Criteria2/1
  [VDDM_Shifter1RCErrRst_flg] -> SR_Latch4/2
  [VDDM_Shifter1CSErrRst_flg] -> SR_Latch7/2
  Switch2/1 -> Test Detection Criteria3/1
  VDDM_Shifter1RCErr_flg/1 -> [VDDM_Shifter1RCErr_flg]
  VDDM_Shifter1CSErr_flg/1 -> [VDDM_Shifter1CSErr_flg]
  [VDDM_Shifter1NoComCFS_flg] -> Logical Operator6/1
  Logical Operator6/1 -> Logical Operator22/4
  [VDDM_Shifter1NoComCFS_flg] -> Logical Operator28/1
  Logical Operator28/1 -> Logical Operator36/4
  Logical Operator39/1 -> Logical Operator15/3
  [DTC_clear_request] -> Logical Operator11/1, Logical Operator39/1
  Logical Operator40/1 -> SR_Latch1/2
  [DTC_clear_request] -> Logical Operator40/2
  [DTC_clear_request] -> Logical Operator77/3
  Logical Operator41/1 -> Logical Operator17/3
  [DTC_clear_request] -> Logical Operator5/1, Logical Operator41/1
  Logical Operator42/1 -> SR_Latch3/2
  [DTC_clear_request] -> Logical Operator42/2
  [DTC_clear_request] -> Logical Operator23/3
  [DTC_clear_request] -> Logical Operator43/1, Logical Operator27/1
  Logical Operator43/1 -> Logical Operator31/3
  [DTC_clear_request] -> Logical Operator44/2
  Logical Operator44/1 -> SR_Latch6/2
  [DTC_clear_request] -> Logical Operator37/3
  [VDDM_Shifter1NoComCFS_flg] -> VDDM_Shifter1NoComCFS_flg/1
  [VDDM_Shifter1RCErrCFS_flg] -> VDDM_Shifter1RCErrCFS_flg/1
  [VDDM_Shifter1CSErrCFS_flg] -> VDDM_Shifter1CSErrCFS_flg/1

== system ddm/DDM/DDM/VMC_DDM/ACC Acceleration Command Error ==
  task_time_s : Inport
  VDDM_FCM2NoComCFS_flg : Inport  Port=2
  VDDM_FCM2RCErrCFS_flg : Inport  Port=3
  VDDM_FCM2CSErrCFS_flg : Inport  Port=4
  VVMC_ADASActive_flg : Inport  Port=5
  No_CAN_BUS_OFF : Inport  Port=6
  VPMM_PowerSta_enum : Inport  Port=7
  VINP_ACCRequireAccel_mps2 : Inport  Port=8
  VINP_ADASACCSta_enum : Inport  Port=9
  DTC_clear_request : Inport  Port=10
  "ACC Acceleration Command Error " : Subsystem
  From5 : From  Commented=on  GotoTag=VDDM_ACCAccelCmdErrDFS_flg
  Terminator : Terminator
  VDDM_ACCAccelCmdErrCFS_flg : Outport
  VDDM_ACCAccelCmdErrDetDTC_raw32 : Outport  Port=2
  wires:
  [VDDM_ACCAccelCmdErrDetDTC_raw32] -> VDDM_ACCAccelCmdErrDetDTC_raw32/1
  "ACC Acceleration Command Error "/2(VDDM_ACCAccelCmdErrDetDTC_raw32) -> [VDDM_ACCAccelCmdErrDetDTC_raw32]
  VINP_ADASACCSta_enum/1 -> [VINP_ADASACCSta_enum]
  [VINP_ADASACCSta_enum] -> "ACC Acceleration Command Error "/9(VINP_ADASACCSta_enum)
  [VVMC_ADASActive_flg] -> "ACC Acceleration Command Error "/5(VVMC_ADASActive_flg)
  VVMC_ADASActive_flg/1 -> [VVMC_ADASActive_flg]
  [task_time_s] -> "ACC Acceleration Command Error "/1(task_time_s)
  task_time_s/1 -> [task_time_s]  "task_time_s"
  [DTC_clear_request] -> "ACC Acceleration Command Error "/10(DTC_clear_request)
  [VINP_ACCRequireAccel_mps2] -> "ACC Acceleration Command Error "/8(VINP_ACCRequireAccel_mps2)
  [VPMM_PowerSta_enum] -> "ACC Acceleration Command Error "/7(VPMM_PowerSta_enum)
  [No_CAN_BUS_OFF] -> "ACC Acceleration Command Error "/6(No_CAN_BUS_OFF)
  [VDDM_FCM2CSErrCFS_flg] -> "ACC Acceleration Command Error "/4(VDDM_FCM2CSErrCFS_flg)
  [VDDM_FCM2RCErrCFS_flg] -> "ACC Acceleration Command Error "/3(VDDM_FCM2RCErrCFS_flg)
  [VDDM_FCM2NoComCFS_flg] -> "ACC Acceleration Command Error "/2(VDDM_FCM2NoComCFS_flg)
  VINP_ACCRequireAccel_mps2/1 -> [VINP_ACCRequireAccel_mps2]
  VDDM_FCM2NoComCFS_flg/1 -> [VDDM_FCM2NoComCFS_flg]
  No_CAN_BUS_OFF/1 -> [No_CAN_BUS_OFF]
  VPMM_PowerSta_enum/1 -> [VPMM_PowerSta_enum]
  DTC_clear_request/1 -> [DTC_clear_request]
  "ACC Acceleration Command Error "/1(VDDM_ACCAccelCmdErrCFS_flg) -> [VDDM_ACCAccelCmdErrCFS_flg]
  From5/1 -> Terminator/1
  [VDDM_ACCAccelCmdErrCFS_flg] -> VDDM_ACCAccelCmdErrCFS_flg/1
  VDDM_FCM2RCErrCFS_flg/1 -> [VDDM_FCM2RCErrCFS_flg]
  VDDM_FCM2CSErrCFS_flg/1 -> [VDDM_FCM2CSErrCFS_flg]

== system ddm/DDM/DDM/VMC_DDM/ACC Malfunction  ==
  task_time_s : Inport
  VDDM_FCMACCSigErrCFS_flg : Inport  Port=2
  VDDM_ACCAccelCmdErrCFS_flg : Inport  Port=3
  VDDM_BMSSigErrCFS_flg : Inport  Port=4
  VDDM_FrMCUSigErrCFS_flg : Inport  Port=5
  VDDM_RrMCUSigErrCFS_flg : Inport  Port=6
  VDDM_CCUSigErrCFS_flg : Inport  Port=7
  VDDM_FCM2NoComCFS_flg : Inport  Port=8
  VDDM_FCM2RCErrCFS_flg : Inport  Port=9
  VDDM_FCM2CSErrCFS_flg : Inport  Port=10
  VDDM_FCM4NoComCFS_flg : Inport  Port=11
  VDDM_FCM4CSErrCFS_flg : Inport  Port=12
  VDDM_ZoneSCPNoComCFS_flg : Inport  Port=13
  VDDM_MCUR1NoComCFS_flg : Inport  Port=14
  VDDM_MCUR1RCErrCFS_flg : Inport  Port=15
  VDDM_MCUR1CSErrCFS_flg : Inport  Port=16
  VDDM_MCUF1NoComCFS_flg : Inport  Port=17
  VDDM_MCUF1RCErrCFS_flg : Inport  Port=18
  VDDM_MCUF1CSErrCFS_flg : Inport  Port=19
  VDDM_ESC7NoComCFS_flg : Inport  Port=20
  VDDM_ESC7RCErrCFS_flg : Inport  Port=21
  VDDM_ESC7CSErrCFS_flg : Inport  Port=22
  VDDM_ESC1NoComCFS_flg : Inport  Port=23
  VDDM_ESC1RCErrCFS_flg : Inport  Port=24
  VDDM_ESC1CSErrCFS_flg : Inport  Port=25
  VDDM_ESC5NoComCFS_flg : Inport  Port=26
  VDDM_ESC5RCErrCFS_flg : Inport  Port=27
  VDDM_ESC5CSErrCFS_flg : Inport  Port=28
  No_CAN1_BUS_OFF : Inport  Port=29
  No_CAN3_BUS_OFF : Inport  Port=30
  No_CAN4_BUS_OFF : Inport  Port=31
  VPMM_PowerSta_enum : Inport  Port=32
  VINP_ZoneSpdCtrlMode_enum : Inport  Port=33
  DTC_clear_request : Inport  Port=34
  "ACC Malfunction " : Subsystem
  From5 : From  Commented=on  GotoTag=VDDM_ACCMalfuncDFS_flg
  Terminator : Terminator
  VDDM_ACCMalfuncCFS_flg : Outport
  VDDM_ACCMalfuncDetDTC_raw32 : Outport  Port=2
  wires:
  [VDDM_ACCMalfuncDetDTC_raw32] -> VDDM_ACCMalfuncDetDTC_raw32/1
  "ACC Malfunction "/2(VDDM_ACCMalfuncDetDTC_raw32) -> [VDDM_ACCMalfuncDetDTC_raw32]
  [VDDM_ZoneSCPNoComCFS_flg] -> "ACC Malfunction "/13(VDDM_ZoneSCPNoComCFS_flg)
  [VDDM_MCUR1RCErrCFS_flg] -> "ACC Malfunction "/15(VDDM_MCUR1RCErrCFS_flg)
  [VINP_ZoneSpdCtrlMode_enum] -> "ACC Malfunction "/33(VINP_ZoneSpdCtrlMode_enum)
  [VDDM_FCM4NoComCFS_flg] -> "ACC Malfunction "/11(VDDM_FCM4NoComCFS_flg)
  [VDDM_ESC5NoComCFS_flg] -> "ACC Malfunction "/26(VDDM_ESC5NoComCFS_flg)
  [VDDM_FCM2RCErrCFS_flg] -> "ACC Malfunction "/9(VDDM_FCM2RCErrCFS_flg)
  [VDDM_FCM2NoComCFS_flg] -> "ACC Malfunction "/8(VDDM_FCM2NoComCFS_flg)
  [VDDM_CCUSigErrCFS_flg] -> "ACC Malfunction "/7(VDDM_CCUSigErrCFS_flg)
  [VDDM_FCM2CSErrCFS_flg] -> "ACC Malfunction "/10(VDDM_FCM2CSErrCFS_flg)
  [VDDM_MCUR1NoComCFS_flg] -> "ACC Malfunction "/14(VDDM_MCUR1NoComCFS_flg)
  [VDDM_MCUF1CSErrCFS_flg] -> "ACC Malfunction "/19(VDDM_MCUF1CSErrCFS_flg)
  [task_time_s] -> "ACC Malfunction "/1(task_time_s)
  [VPMM_PowerSta_enum] -> "ACC Malfunction "/32(VPMM_PowerSta_enum)
  [VDDM_FCMACCSigErrCFS_flg] -> "ACC Malfunction "/2(VDDM_FCMACCSigErrCFS_flg)
  [No_CAN1_BUS_OFF] -> "ACC Malfunction "/29(No_CAN1_BUS_OFF)
  [VDDM_ESC1CSErrCFS_flg] -> "ACC Malfunction "/25(VDDM_ESC1CSErrCFS_flg)
  [VDDM_ESC1NoComCFS_flg] -> "ACC Malfunction "/23(VDDM_ESC1NoComCFS_flg)
  [VDDM_ESC5RCErrCFS_flg] -> "ACC Malfunction "/27(VDDM_ESC5RCErrCFS_flg)
  [VDDM_ESC5CSErrCFS_flg] -> "ACC Malfunction "/28(VDDM_ESC5CSErrCFS_flg)
  [VDDM_ESC7NoComCFS_flg] -> "ACC Malfunction "/20(VDDM_ESC7NoComCFS_flg)
  [VDDM_ESC7RCErrCFS_flg] -> "ACC Malfunction "/21(VDDM_ESC7RCErrCFS_flg)
  [VDDM_ESC1RCErrCFS_flg] -> "ACC Malfunction "/24(VDDM_ESC1RCErrCFS_flg)
  [VDDM_FCM4CSErrCFS_flg] -> "ACC Malfunction "/12(VDDM_FCM4CSErrCFS_flg)
  [VDDM_ESC7CSErrCFS_flg] -> "ACC Malfunction "/22(VDDM_ESC7CSErrCFS_flg)
  [VDDM_MCUF1RCErrCFS_flg] -> "ACC Malfunction "/18(VDDM_MCUF1RCErrCFS_flg)
  [VDDM_ACCAccelCmdErrCFS_flg] -> "ACC Malfunction "/3(VDDM_ACCAccelCmdErrCFS_flg)
  [DTC_clear_request] -> "ACC Malfunction "/34(DTC_clear_request)
  [VDDM_FrMCUSigErrCFS_flg] -> "ACC Malfunction "/5(VDDM_FrMCUSigErrCFS_flg)
  [No_CAN4_BUS_OFF] -> "ACC Malfunction "/31(No_CAN4_BUS_OFF)
  [VDDM_MCUF1NoComCFS_flg] -> "ACC Malfunction "/17(VDDM_MCUF1NoComCFS_flg)
  [VDDM_BMSSigErrCFS_flg] -> "ACC Malfunction "/4(VDDM_BMSSigErrCFS_flg)
  [VDDM_RrMCUSigErrCFS_flg] -> "ACC Malfunction "/6(VDDM_RrMCUSigErrCFS_flg)
  [VDDM_MCUR1CSErrCFS_flg] -> "ACC Malfunction "/16(VDDM_MCUR1CSErrCFS_flg)
  [No_CAN3_BUS_OFF] -> "ACC Malfunction "/30(No_CAN3_BUS_OFF)
  DTC_clear_request/1 -> [DTC_clear_request]
  No_CAN4_BUS_OFF/1 -> [No_CAN4_BUS_OFF]
  No_CAN3_BUS_OFF/1 -> [No_CAN3_BUS_OFF]
  VDDM_ESC5NoComCFS_flg/1 -> [VDDM_ESC5NoComCFS_flg]
  VDDM_ESC5RCErrCFS_flg/1 -> [VDDM_ESC5RCErrCFS_flg]
  VDDM_ESC5CSErrCFS_flg/1 -> [VDDM_ESC5CSErrCFS_flg]
  VDDM_MCUR1CSErrCFS_flg/1 -> [VDDM_MCUR1CSErrCFS_flg]
  VDDM_MCUR1RCErrCFS_flg/1 -> [VDDM_MCUR1RCErrCFS_flg]
  VDDM_MCUR1NoComCFS_flg/1 -> [VDDM_MCUR1NoComCFS_flg]
  VDDM_MCUF1NoComCFS_flg/1 -> [VDDM_MCUF1NoComCFS_flg]
  VDDM_MCUF1RCErrCFS_flg/1 -> [VDDM_MCUF1RCErrCFS_flg]
  VDDM_MCUF1CSErrCFS_flg/1 -> [VDDM_MCUF1CSErrCFS_flg]
  VDDM_ESC1CSErrCFS_flg/1 -> [VDDM_ESC1CSErrCFS_flg]
  VDDM_ESC1RCErrCFS_flg/1 -> [VDDM_ESC1RCErrCFS_flg]
  VDDM_ESC1NoComCFS_flg/1 -> [VDDM_ESC1NoComCFS_flg]
  VDDM_ESC7NoComCFS_flg/1 -> [VDDM_ESC7NoComCFS_flg]
  VDDM_ESC7RCErrCFS_flg/1 -> [VDDM_ESC7RCErrCFS_flg]
  VDDM_ESC7CSErrCFS_flg/1 -> [VDDM_ESC7CSErrCFS_flg]
  VDDM_FCM2CSErrCFS_flg/1 -> [VDDM_FCM2CSErrCFS_flg]
  VDDM_FCM2RCErrCFS_flg/1 -> [VDDM_FCM2RCErrCFS_flg]
  VDDM_FCM2NoComCFS_flg/1 -> [VDDM_FCM2NoComCFS_flg]
  VDDM_FCM4NoComCFS_flg/1 -> [VDDM_FCM4NoComCFS_flg]
  VDDM_FCM4CSErrCFS_flg/1 -> [VDDM_FCM4CSErrCFS_flg]
  VDDM_ZoneSCPNoComCFS_flg/1 -> [VDDM_ZoneSCPNoComCFS_flg]
  VDDM_CCUSigErrCFS_flg/1 -> [VDDM_CCUSigErrCFS_flg]
  VDDM_RrMCUSigErrCFS_flg/1 -> [VDDM_RrMCUSigErrCFS_flg]
  VDDM_FrMCUSigErrCFS_flg/1 -> [VDDM_FrMCUSigErrCFS_flg]
  task_time_s/1 -> [task_time_s]  "task_time_s"
  VINP_ZoneSpdCtrlMode_enum/1 -> [VINP_ZoneSpdCtrlMode_enum]
  VDDM_FCMACCSigErrCFS_flg/1 -> [VDDM_FCMACCSigErrCFS_flg]
  No_CAN1_BUS_OFF/1 -> [No_CAN1_BUS_OFF]
  VPMM_PowerSta_enum/1 -> [VPMM_PowerSta_enum]
  "ACC Malfunction "/1(VDDM_ACCMalfuncCFS_flg) -> [VDDM_ACCMalfuncCFS_flg]
  From5/1 -> Terminator/1
  [VDDM_ACCMalfuncCFS_flg] -> VDDM_ACCMalfuncCFS_flg/1
  VDDM_ACCAccelCmdErrCFS_flg/1 -> [VDDM_ACCAccelCmdErrCFS_flg]
  VDDM_BMSSigErrCFS_flg/1 -> [VDDM_BMSSigErrCFS_flg]

== system ddm/DDM/DDM/VMC_DDM/BMS Signal Error  ==
  task_time_s : Inport
  VDDM_C3BMS6LCCFS_flg : Inport  Port=2
  VDDM_C3BMS6RCCFS_flg : Inport  Port=3
  VDDM_C3BMS6CSCFS_flg : Inport  Port=4
  No_CAN_BUS_OFF : Inport  Port=5
  VPMM_PowerSta_enum : Inport  Port=6
  VINP_BMSWarn8_flg : Inport  Port=7
  VINP_BMSWarn7_flg : Inport  Port=8
  VINP_BMSWarn6_flg : Inport  Port=9
  VINP_BMSWarn5_flg : Inport  Port=10
  VINP_BMSWarn4_flg : Inport  Port=11
  DTC_clear_request : Inport  Port=12
  "BMS Signal Error " : Subsystem
  From5 : From  Commented=on  GotoTag=VDDM_BMSSigErrDFS_flg
  Terminator : Terminator
  VDDM_BMSSigErrCFS_flg : Outport
  VDDM_BMSSigErrDetDTC_raw32 : Outport  Port=2
  wires:
  [VDDM_BMSSigErrDetDTC_raw32] -> VDDM_BMSSigErrDetDTC_raw32/1
  "BMS Signal Error "/2(VDDM_BMSSigErrDetDTC_raw32) -> [VDDM_BMSSigErrDetDTC_raw32]
  [task_time_s] -> "BMS Signal Error "/1(task_time_s)
  task_time_s/1 -> [task_time_s]  "task_time_s"
  [DTC_clear_request] -> "BMS Signal Error "/12(DTC_clear_request)
  [VINP_BMSWarn4_flg] -> "BMS Signal Error "/11(VINP_BMSWarn4_flg)
  [VINP_BMSWarn5_flg] -> "BMS Signal Error "/10(VINP_BMSWarn5_flg)
  [VINP_BMSWarn6_flg] -> "BMS Signal Error "/9(VINP_BMSWarn6_flg)
  [VINP_BMSWarn7_flg] -> "BMS Signal Error "/8(VINP_BMSWarn7_flg)
  [VINP_BMSWarn8_flg] -> "BMS Signal Error "/7(VINP_BMSWarn8_flg)
  [VPMM_PowerSta_enum] -> "BMS Signal Error "/6(VPMM_PowerSta_enum)
  [No_CAN_BUS_OFF] -> "BMS Signal Error "/5(No_CAN_BUS_OFF)
  [VDDM_C3BMS6CSCFS_flg] -> "BMS Signal Error "/4(VDDM_C3BMS6CSCFS_flg)
  [VDDM_C3BMS6RCCFS_flg] -> "BMS Signal Error "/3(VDDM_C3BMS6RCCFS_flg)
  [VDDM_C3BMS6LCCFS_flg] -> "BMS Signal Error "/2(VDDM_C3BMS6LCCFS_flg)
  VINP_BMSWarn4_flg/1 -> [VINP_BMSWarn4_flg]
  VINP_BMSWarn6_flg/1 -> [VINP_BMSWarn6_flg]
  VINP_BMSWarn5_flg/1 -> [VINP_BMSWarn5_flg]
  VINP_BMSWarn7_flg/1 -> [VINP_BMSWarn7_flg]
  VINP_BMSWarn8_flg/1 -> [VINP_BMSWarn8_flg]
  VDDM_C3BMS6LCCFS_flg/1 -> [VDDM_C3BMS6LCCFS_flg]
  No_CAN_BUS_OFF/1 -> [No_CAN_BUS_OFF]
  VPMM_PowerSta_enum/1 -> [VPMM_PowerSta_enum]
  DTC_clear_request/1 -> [DTC_clear_request]
  "BMS Signal Error "/1(VDDM_BMSSigErrCFS_flg) -> [VDDM_BMSSigErrCFS_flg]
  From5/1 -> Terminator/1
  [VDDM_BMSSigErrCFS_flg] -> VDDM_BMSSigErrCFS_flg/1
  VDDM_C3BMS6RCCFS_flg/1 -> [VDDM_C3BMS6RCCFS_flg]
  VDDM_C3BMS6CSCFS_flg/1 -> [VDDM_C3BMS6CSCFS_flg]

== system ddm/DDM/DDM/VMC_DDM/CC Malfunction  ==
  task_time_s : Inport
  VDDM_BMSSigErrCFS_flg : Inport  Port=2
  VDDM_FrMCUSigErrCFS_flg : Inport  Port=3
  VDDM_RrMCUSigErrCFS_flg : Inport  Port=4
  VDDM_CCUSigErrCFS_flg : Inport  Port=5
  VDDM_ZoneSCPNoComCFS_flg : Inport  Port=6
  VDDM_MCUR1NoComCFS_flg : Inport  Port=7
  VDDM_MCUR1RCErrCFS_flg : Inport  Port=8
  VDDM_MCUR1CSErrCFS_flg : Inport  Port=9
  VDDM_MCUF1NoComCFS_flg : Inport  Port=10
  VDDM_MCUF1RCErrCFS_flg : Inport  Port=11
  VDDM_MCUF1CSErrCFS_flg : Inport  Port=12
  VDDM_ESC7NoComCFS_flg : Inport  Port=13
  VDDM_ESC7RCErrCFS_flg : Inport  Port=14
  VDDM_ESC7CSErrCFS_flg : Inport  Port=15
  VDDM_ESC1NoComCFS_flg : Inport  Port=16
  VDDM_ESC1RCErrCFS_flg : Inport  Port=17
  VDDM_ESC1CSErrCFS_flg : Inport  Port=18
  VDDM_ESC5NoComCFS_flg : Inport  Port=19
  VDDM_ESC5RCErrCFS_flg : Inport  Port=20
  VDDM_ESC5CSErrCFS_flg : Inport  Port=21
  No_CAN1_BUS_OFF : Inport  Port=22
  No_CAN3_BUS_OFF : Inport  Port=23
  No_CAN4_BUS_OFF : Inport  Port=24
  VPMM_PowerSta_enum : Inport  Port=25
  VINP_ZoneSpdCtrlMode_enum : Inport  Port=26
  DTC_clear_request : Inport  Port=27
  "CC Malfunction " : Subsystem
  From5 : From  Commented=on  GotoTag=VDDM_CCMalfuncDFS_flg
  Terminator : Terminator
  VDDM_CCMalfuncCFS_flg : Outport
  VDDM_CCMalfuncDetDTC_raw32 : Outport  Port=2
  wires:
  [VDDM_CCMalfuncDetDTC_raw32] -> VDDM_CCMalfuncDetDTC_raw32/1
  "CC Malfunction "/2(VDDM_CCMalfuncDetDTC_raw32) -> [VDDM_CCMalfuncDetDTC_raw32]
  [DTC_clear_request] -> "CC Malfunction "/27(DTC_clear_request)
  [VINP_ZoneSpdCtrlMode_enum] -> "CC Malfunction "/26(VINP_ZoneSpdCtrlMode_enum)
  [VPMM_PowerSta_enum] -> "CC Malfunction "/25(VPMM_PowerSta_enum)
  [No_CAN4_BUS_OFF] -> "CC Malfunction "/24(No_CAN4_BUS_OFF)
  [No_CAN3_BUS_OFF] -> "CC Malfunction "/23(No_CAN3_BUS_OFF)
  [No_CAN1_BUS_OFF] -> "CC Malfunction "/22(No_CAN1_BUS_OFF)
  [VDDM_ESC5CSErrCFS_flg] -> "CC Malfunction "/21(VDDM_ESC5CSErrCFS_flg)
  [VDDM_ESC5RCErrCFS_flg] -> "CC Malfunction "/20(VDDM_ESC5RCErrCFS_flg)
  [VDDM_ESC5NoComCFS_flg] -> "CC Malfunction "/19(VDDM_ESC5NoComCFS_flg)
  [VDDM_ESC1CSErrCFS_flg] -> "CC Malfunction "/18(VDDM_ESC1CSErrCFS_flg)
  [VDDM_ESC1RCErrCFS_flg] -> "CC Malfunction "/17(VDDM_ESC1RCErrCFS_flg)
  [VDDM_ESC1NoComCFS_flg] -> "CC Malfunction "/16(VDDM_ESC1NoComCFS_flg)
  [VDDM_ESC7CSErrCFS_flg] -> "CC Malfunction "/15(VDDM_ESC7CSErrCFS_flg)
  [VDDM_ESC7RCErrCFS_flg] -> "CC Malfunction "/14(VDDM_ESC7RCErrCFS_flg)
  [VDDM_ESC7NoComCFS_flg] -> "CC Malfunction "/13(VDDM_ESC7NoComCFS_flg)
  [VDDM_MCUF1CSErrCFS_flg] -> "CC Malfunction "/12(VDDM_MCUF1CSErrCFS_flg)
  [VDDM_MCUF1RCErrCFS_flg] -> "CC Malfunction "/11(VDDM_MCUF1RCErrCFS_flg)
  [VDDM_MCUF1NoComCFS_flg] -> "CC Malfunction "/10(VDDM_MCUF1NoComCFS_flg)
  [VDDM_MCUR1CSErrCFS_flg] -> "CC Malfunction "/9(VDDM_MCUR1CSErrCFS_flg)
  [VDDM_MCUR1RCErrCFS_flg] -> "CC Malfunction "/8(VDDM_MCUR1RCErrCFS_flg)
  [VDDM_MCUR1NoComCFS_flg] -> "CC Malfunction "/7(VDDM_MCUR1NoComCFS_flg)
  [VDDM_ZoneSCPNoComCFS_flg] -> "CC Malfunction "/6(VDDM_ZoneSCPNoComCFS_flg)
  [VDDM_CCUSigErrCFS_flg] -> "CC Malfunction "/5(VDDM_CCUSigErrCFS_flg)
  [VDDM_RrMCUSigErrCFS_flg] -> "CC Malfunction "/4(VDDM_RrMCUSigErrCFS_flg)
  [VDDM_FrMCUSigErrCFS_flg] -> "CC Malfunction "/3(VDDM_FrMCUSigErrCFS_flg)
  [VDDM_BMSSigErrCFS_flg] -> "CC Malfunction "/2(VDDM_BMSSigErrCFS_flg)
  [task_time_s] -> "CC Malfunction "/1(task_time_s)
  DTC_clear_request/1 -> [DTC_clear_request]
  No_CAN4_BUS_OFF/1 -> [No_CAN4_BUS_OFF]
  No_CAN3_BUS_OFF/1 -> [No_CAN3_BUS_OFF]
  VDDM_ESC5NoComCFS_flg/1 -> [VDDM_ESC5NoComCFS_flg]
  VDDM_ESC5RCErrCFS_flg/1 -> [VDDM_ESC5RCErrCFS_flg]
  VDDM_ESC5CSErrCFS_flg/1 -> [VDDM_ESC5CSErrCFS_flg]
  VDDM_MCUR1CSErrCFS_flg/1 -> [VDDM_MCUR1CSErrCFS_flg]
  VDDM_MCUR1RCErrCFS_flg/1 -> [VDDM_MCUR1RCErrCFS_flg]
  VDDM_MCUR1NoComCFS_flg/1 -> [VDDM_MCUR1NoComCFS_flg]
  VDDM_MCUF1NoComCFS_flg/1 -> [VDDM_MCUF1NoComCFS_flg]
  VDDM_MCUF1RCErrCFS_flg/1 -> [VDDM_MCUF1RCErrCFS_flg]
  VDDM_MCUF1CSErrCFS_flg/1 -> [VDDM_MCUF1CSErrCFS_flg]
  VDDM_ESC1CSErrCFS_flg/1 -> [VDDM_ESC1CSErrCFS_flg]
  VDDM_ESC1RCErrCFS_flg/1 -> [VDDM_ESC1RCErrCFS_flg]
  VDDM_ESC1NoComCFS_flg/1 -> [VDDM_ESC1NoComCFS_flg]
  VDDM_ESC7NoComCFS_flg/1 -> [VDDM_ESC7NoComCFS_flg]
  VDDM_ESC7RCErrCFS_flg/1 -> [VDDM_ESC7RCErrCFS_flg]
  VDDM_ESC7CSErrCFS_flg/1 -> [VDDM_ESC7CSErrCFS_flg]
  VDDM_ZoneSCPNoComCFS_flg/1 -> [VDDM_ZoneSCPNoComCFS_flg]
  VDDM_CCUSigErrCFS_flg/1 -> [VDDM_CCUSigErrCFS_flg]
  VDDM_RrMCUSigErrCFS_flg/1 -> [VDDM_RrMCUSigErrCFS_flg]
  VDDM_FrMCUSigErrCFS_flg/1 -> [VDDM_FrMCUSigErrCFS_flg]
  task_time_s/1 -> [task_time_s]  "task_time_s"
  VINP_ZoneSpdCtrlMode_enum/1 -> [VINP_ZoneSpdCtrlMode_enum]
  No_CAN1_BUS_OFF/1 -> [No_CAN1_BUS_OFF]
  VPMM_PowerSta_enum/1 -> [VPMM_PowerSta_enum]
  "CC Malfunction "/1(VDDM_CCMalfuncCFS_flg) -> [VDDM_CCMalfuncCFS_flg]
  From5/1 -> Terminator/1
  [VDDM_CCMalfuncCFS_flg] -> VDDM_CCMalfuncCFS_flg/1
  VDDM_BMSSigErrCFS_flg/1 -> [VDDM_BMSSigErrCFS_flg]
